simulink library "pressure_drop_calculated_data_water"  (R2018b)
settings: Solver=ode45  StartTime=0.0  StopTime=10.0  RelTol=1e-3  EnableMultiTasking=on
undefined symbols (not defined in the file): acol
settings Model: Creator=lena.frank  LastModifiedBy=drhf
settings DataIOCC: LimitDataPoints=on  SaveFormat=Array  SignalLoggingSaveFormat=ModelDataLogs
settings OptimizationCC: ExpressionDepthLimit=2147483647  LifeSpan=inf
settings DebuggingCC: UnderspecifiedInitializationDetection=Classic  MergeDetectMultiDrivingBlocksExec=none  SolverPrmCheckMsg=warning  FcnCallInpInsideContextMsg=warning  StateNameClashWarn=warning  SFUnexpectedBacktrackingDiag=warning  SFNoUnconditionalDefaultTransitionDiag=warning  SFExecutionAtInitializationDiag=none
settings HardwareCC: ProdBitPerPointer=32  ProdBitPerSizeT=32  ProdBitPerPtrDiffT=32  ProdLargestAtomicFloat=None  ProdIntDivRoundTo=Undefined  ProdEndianess=Unspecified  ProdWordSize=32  ProdHWDeviceType=32-bit Generic
settings ModelReferenceCC: PropagateSignalLabelsOutOfModel=off
settings SFSimCC: SimUseLocalCustomCode=off
settings RTWCC: RTWUseLocalCustomCode=off
settings CodeAppCC: StateflowObjectComments=on
settings GRTTargetCC: TargetLangStandard=C89/C90 (ANSI)  GeneratePreprocessorConditionals=Disable all  CombineOutputUpdateFcns=off  GRTInterface=on
settings ConfigComp: CovMetricSettings=dw  CovHtmlReporting=on  CovSaveCumulativeToWorkspaceVar=on  CovSaveSingleToWorkspaceVar=on  CovExternalEMLEnable=off

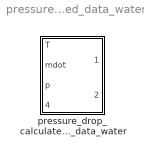
== system pressure_drop_calculated_data_water ==
  pressure_drop_calculated_data_water : Subsystem  mask(pressure drop for header - riser, fluid water){aonecol=1.96, acol=acol}
      mask prompts: aonecol "surface of one collector element [m²]"; acol "total surface of array (DO NOT CHANGE)"
      mask help:
      | This block interpolates the pressure drop of a collector for a usual header riser- arrangement. The number of risers (= number of absorber fins) is 10 per m². The inner diameter of the riser is 6 mm, of the header 20 mm. Fluid in the collector is water. An equation of Dunkle and Davey ("Flow distribution in absorber banks", ISES Conference, 1970) is used. See colpdrop in the manual or type "help colpdrop" on the command line for more information.
      | Set "surface of one collector" to the surface of one collector for a parallel arrangement of collectors. Set it to the surface of the array "acol" to model a series arrangement.
      mask Help: web(fullfile(path_carnot('help'),'pressure_drop_calculated_for_header_riser_water.html'),'-helpbrowser')

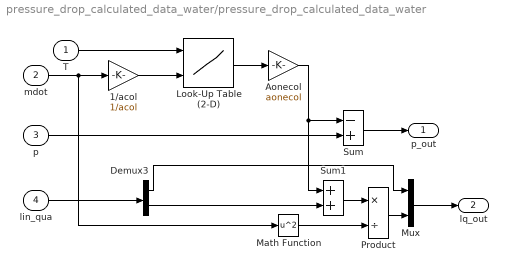
== system pressure_drop_calculated_data_water/pressure_drop_calculated_data_water ==
  T : Inport
  mdot : Inport  Port=2
  p : Inport  Port=3
  lin_qua : Inport  Port=4
  1/acol : Gain  Gain=1/acol  SaturateOnIntegerOverflow=on  OutDataTypeStr=Inherit: Same as input  ParamDataTypeStr=Inherit: Same as input
  Aonecol : Gain  Gain=aonecol  SaturateOnIntegerOverflow=on  OutDataTypeStr=Inherit: Same as input  ParamDataTypeStr=Inherit: Same as input
  Demux3 : Demux  Outputs=2
  Look-Up Table (2-D) : Lookup2D  RowIndex=0:50:200  ColumnIndex=0:0.01:0.05  Table="[0 121.8750 261.8368 419.7212 595.443 788.9438; 0 44.3145 106.6853 186.9531 285.0355 400.8755; 0 29.8974 78.2964 145.0362 230.0334 333.2306; 0 24.2577 67.8077 130.4839 212.2001 312.8971; 0  21.7174 64.2104 127.3018 210.8995 314.9402]"  SaturateOnIntegerOverflow=on  InputSameDT=on
  Math Function : Math  Operator=square  SaturateOnIntegerOverflow=on
  Mux : Mux  Inputs=2
  Product : Product  Inputs=*/  SaturateOnIntegerOverflow=on  InputSameDT=on  OutDataTypeStr=Inherit: Same as first input
  Sum : Sum  Inputs=-+  SaturateOnIntegerOverflow=on  InputSameDT=on  OutDataTypeStr=Inherit: Same as first input
  Sum1 : Sum  SaturateOnIntegerOverflow=on  InputSameDT=on  OutDataTypeStr=Inherit: Same as first input
  p_out : Outport
  lq_out : Outport  Port=2
  wires:
  Aonecol/1 -> Sum1/1, Sum/1
  p/1 -> Sum/2
  Sum/1 -> p_out/1
  Demux3/1 -> Mux/1
  Mux/1 -> lq_out/1
  Product/1 -> Mux/2
  Math Function/1 -> Product/2
  Sum1/1 -> Product/1
  Demux3/2 -> Sum1/2
  lin_qua/1 -> Demux3/1
  mdot/1 -> Math Function/1, 1/acol/1
  1/acol/1 -> Look-Up Table (2-D)/2
  T/1 -> Look-Up Table (2-D)/1
  Look-Up Table (2-D)/1 -> Aonecol/1
